simulink model "wiper_prpject_second_way_edit"  (R2021a)
settings: Solver=FixedStepAuto  StartTime=0.0  StopTime=inf  FixedStep=0.01  RelTol=1e-3
model workspace (MAT data in the model file):
  Sig = Simulink.Signal
  Sig.DataType = 'auto'
  Sig.Dimensions = -1
  Sig.DimensionsMode = 'auto'
  Sig.Complexity = 'auto'
  Sig.SampleTime = -1
  Sig.SamplingMode = 'auto'
  x_data_table = Simulink.Parameter
  x_data_table.Value = [0 1 2 3 4 5 6 7]
  x_data_table.DataType = 'auto'
  x_data_table.Dimensions = [1 8]
  y_data_table = Simulink.Parameter
  y_data_table.Value = [0 0.4 0.45 0.5 0.55 0.6 0.65 0.75]
  y_data_table.DataType = 'auto'
  y_data_table.Dimensions = [1 8]
undefined symbols (not defined in the file): speed_mode
libraries: simulink x2
settings Model: EnablePacing=on  PacingRate=0.250000  Creator=Beshary  LastModifiedBy=Beshary
settings OptimizationCC: DefaultUnderspecifiedDataType=single

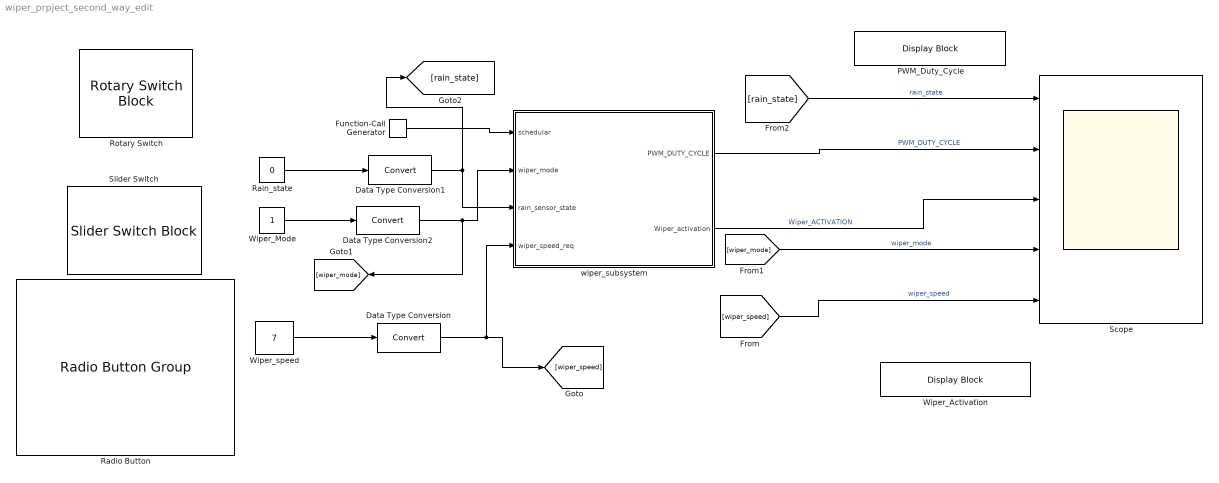
== system wiper_prpject_second_way_edit ==
  Data Type Conversion : DataTypeConversion
  Data Type Conversion1 : DataTypeConversion
  Data Type Conversion2 : DataTypeConversion
  Function-Call Generator : simulink/Ports & Subsystems/Function-Call Generator  sample_time=0.01  numberOfIterations=1  DisallowWideOutput=off
  PWM_Duty_Cycle : DisplayBlock  Format=short  Transparency=1
  Radio Button : RadioButtonGroup  SelectedLabel=speed_mode(7)  ButtonGroupName=Group
      settings: Values={{'speed_mode(0)', 'speed_mode(1)', 'speed_mode(2)', 'speed_mode(3)', 'speed_mode(4)', 'speed_mode(5)', 'speed_mode(6)', 'speed_mode(7)'}, [0 1 2 3 4 5 6 7]}
  Rain_state : Constant  Value=0
  Rotary Switch : RotarySwitchBlock
      settings: Values={{'Off', 'Aut', 'LoSpd', 'HiSpod'}, [0 1 2 3]}
  Scope : Scope  NumInputPorts=5
  Slider Switch : SliderSwitchBlock
      settings: Values={{'Normal', 'Error'}, [0 1]}
  Wiper_Activation : DisplayBlock  Format=short  Transparency=1
  Wiper_Mode : Constant
  Wiper_speed : Constant  Value=7  OutDataTypeStr=int8
  wiper_subsystem : Subsystem
  wires:
  Data Type Conversion2/1 -> wiper_subsystem/2(wiper_mode), [wiper_mode]
  [rain_state] -> Scope/1  "rain_state"
  Data Type Conversion/1 -> [wiper_speed], wiper_subsystem/4(wiper_speed_req)
  wiper_subsystem/1(PWM_DUTY_CYCLE) -> Scope/2  "PWM_DUTY_CYCLE"
  wiper_subsystem/2(Wiper_activation) -> Scope/3  "Wiper_ACTIVATION"
  Function-Call Generator/1 -> wiper_subsystem/1(schedular)
  [wiper_mode] -> Scope/4  "wiper_mode"
  [wiper_speed] -> Scope/5  "wiper_speed"
  Data Type Conversion1/1 -> wiper_subsystem/3(rain_sensor_state), [rain_state]
  Wiper_Mode/1 -> Data Type Conversion2/1
  Wiper_speed/1 -> Data Type Conversion/1
  Rain_state/1 -> Data Type Conversion1/1

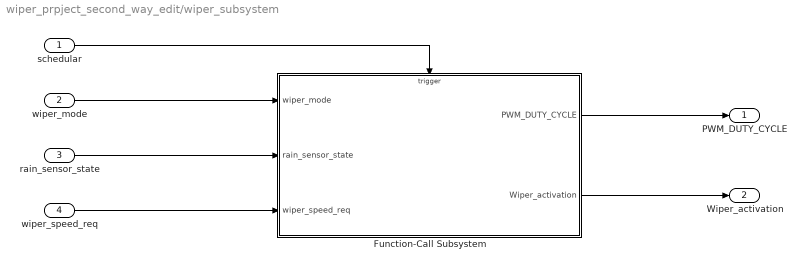
== system wiper_prpject_second_way_edit/wiper_subsystem ==
  schedular : Inport
  wiper_mode : Inport  Port=2  OutDataTypeStr=uint16
  rain_sensor_state : Inport  Port=3  OutDataTypeStr=boolean
  wiper_speed_req : Inport  Port=4  OutDataTypeStr=uint8
  Function-Call Subsystem : Subsystem  TreatAsAtomicUnit=on
  PWM_DUTY_CYCLE : Outport  OutDataTypeStr=single
  Wiper_activation : Outport  Port=2  OutDataTypeStr=boolean
  wires:
  schedular/1 -> Function-Call Subsystem/Trigger
  wiper_mode/1 -> Function-Call Subsystem/1(wiper_mode)
  rain_sensor_state/1 -> Function-Call Subsystem/2(rain_sensor_state)
  wiper_speed_req/1 -> Function-Call Subsystem/3(wiper_speed_req)
  Function-Call Subsystem/1(PWM_DUTY_CYCLE) -> PWM_DUTY_CYCLE/1
  Function-Call Subsystem/2(Wiper_activation) -> Wiper_activation/1

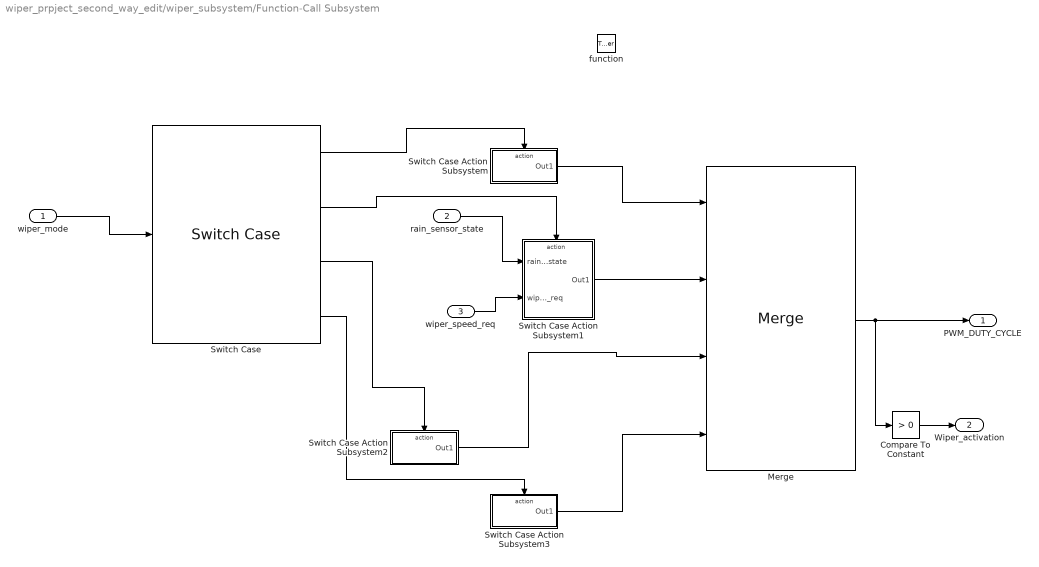
== system wiper_prpject_second_way_edit/wiper_subsystem/Function-Call Subsystem ==
  wiper_mode : Inport  OutDataTypeStr=uint16
  rain_sensor_state : Inport  Port=2  OutDataTypeStr=boolean
  wiper_speed_req : Inport  Port=3
  function : TriggerPort  TriggerType=function-call  VariantControl=(inherit)
  Compare To Constant : simulink/Logic and Bit Operations/Compare To Constant  relop=>  const=0  OutDataTypeStr=boolean
  Merge : Merge  Inputs=4
  Switch Case : SwitchCase  CaseConditions={0,1,2,3}  ShowDefaultCase=off
  Switch Case Action Subsystem : Subsystem  TreatAsAtomicUnit=on
  Switch Case Action Subsystem1 : Subsystem  TreatAsAtomicUnit=on
  Switch Case Action Subsystem2 : Subsystem  TreatAsAtomicUnit=on
  Switch Case Action Subsystem3 : Subsystem  TreatAsAtomicUnit=on
  PWM_DUTY_CYCLE : Outport
  Wiper_activation : Outport  Port=2
  wires:
  Switch Case/1 -> Switch Case Action Subsystem/Action
  Switch Case/2 -> Switch Case Action Subsystem1/Action
  Switch Case/3 -> Switch Case Action Subsystem2/Action
  Switch Case/4 -> Switch Case Action Subsystem3/Action
  wiper_mode/1 -> Switch Case/1
  Switch Case Action Subsystem/1(Out1) -> Merge/1
  Switch Case Action Subsystem1/1(Out1) -> Merge/2
  Switch Case Action Subsystem2/1(Out1) -> Merge/3
  Switch Case Action Subsystem3/1(Out1) -> Merge/4
  Merge/1 -> Compare To Constant/1, PWM_DUTY_CYCLE/1
  rain_sensor_state/1 -> Switch Case Action Subsystem1/1(rain_sensor_state)
  wiper_speed_req/1 -> Switch Case Action Subsystem1/2(wiper_speed_req)
  Compare To Constant/1 -> Wiper_activation/1

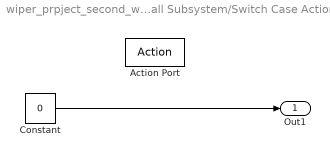
== system wiper_prpject_second_way_edit/wiper_subsystem/Function-Call Subsystem/Switch Case Action Subsystem ==
  Action Port : ActionPort  ActionPortLabel=case [ 0 ]:
  Constant : Constant  Value=0  OutDataTypeStr=single
  Out1 : Outport  OutDataTypeStr=single
  wires:
  Constant/1 -> Out1/1

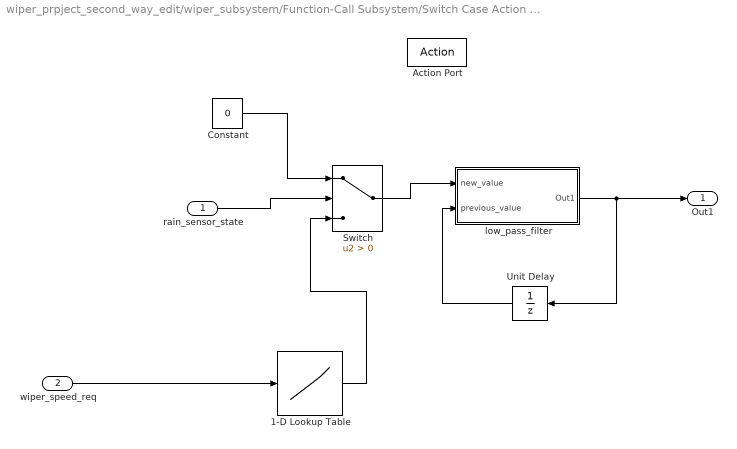
== system wiper_prpject_second_way_edit/wiper_subsystem/Function-Call Subsystem/Switch Case Action Subsystem1 ==
  rain_sensor_state : Inport  OutDataTypeStr=boolean
  wiper_speed_req : Inport  Port=2
  Action Port : ActionPort  ActionPortLabel=case [ 1 ]:
  1-D Lookup Table : Lookup_n-D  NumberOfTableDimensions=1  BreakpointsForDimension1=x_data_table  Table=y_data_table  TableDataTypeStr=single  InterpMethod=Nearest  InternalRulePriority=Speed  OutDataTypeStr=single  RndMeth=Simplest  InputSameDT=on
  Constant : Constant  Value=0  OutDataTypeStr=single
  Switch : Switch  Criteria=u2 > Threshold
  Unit Delay : UnitDelay  SampleTime=-1  HasFrameUpgradeWarning=on
  low_pass_filter : Subsystem
  Out1 : Outport  OutDataTypeStr=single
  wires:
  rain_sensor_state/1 -> Switch/2
  Constant/1 -> Switch/1
  Switch/1 -> low_pass_filter/1(new_value)
  wiper_speed_req/1 -> 1-D Lookup Table/1
  low_pass_filter/1(Out1) -> Unit Delay/1, Out1/1
  1-D Lookup Table/1 -> Switch/3
  Unit Delay/1 -> low_pass_filter/2(previous_value)

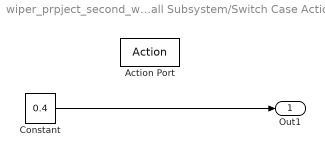
== system wiper_prpject_second_way_edit/wiper_subsystem/Function-Call Subsystem/Switch Case Action Subsystem2 ==
  Action Port : ActionPort  ActionPortLabel=case [ 2 ]:
  Constant : Constant  Value=0.4  OutDataTypeStr=single
  Out1 : Outport  OutDataTypeStr=single
  wires:
  Constant/1 -> Out1/1

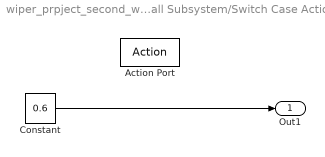
== system wiper_prpject_second_way_edit/wiper_subsystem/Function-Call Subsystem/Switch Case Action Subsystem3 ==
  Action Port : ActionPort  ActionPortLabel=case [ 3 ]:
  Constant : Constant  Value=0.6  OutDataTypeStr=single
  Out1 : Outport  OutDataTypeStr=single
  wires:
  Constant/1 -> Out1/1

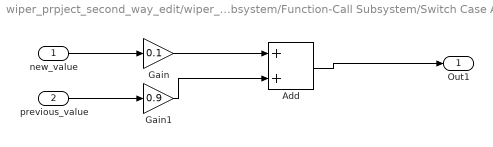
== system wiper_prpject_second_way_edit/wiper_subsystem/Function-Call Subsystem/Switch Case Action Subsystem1/low_pass_filter ==
  new_value : Inport  OutDataTypeStr=single
  previous_value : Inport  Port=2
  Add : Sum  AccumDataTypeStr=single  OutDataTypeStr=single
  Gain : Gain  Gain=0.1  ParamDataTypeStr=single  OutDataTypeStr=single
  Gain1 : Gain  Gain=0.9
  Out1 : Outport  OutDataTypeStr=single
  wires:
  new_value/1 -> Gain/1
  previous_value/1 -> Gain1/1
  Gain1/1 -> Add/2
  Gain/1 -> Add/1
  Add/1 -> Out1/1
